simulink model "model_steadystate_pmsm"  (R2022a)
settings: Solver=ode4  StartTime=0.0  StopTime=1  FixedStep=1e-4  RelTol=1e-3
PreLoadFcn:
  | P = 2; %number of poles
settings Model: Creator=samee  LastModifiedBy=samee

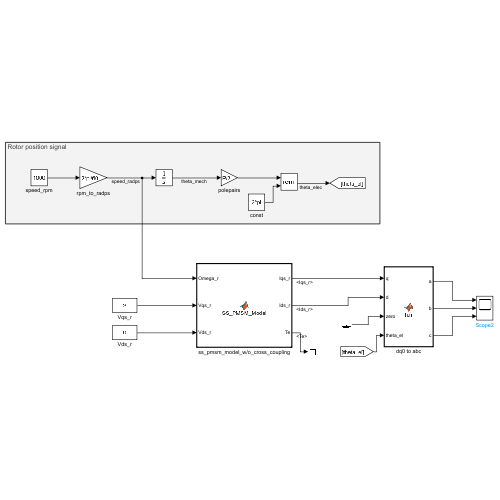
[thumbnail: Simulink's stored preview of the top-level diagram]
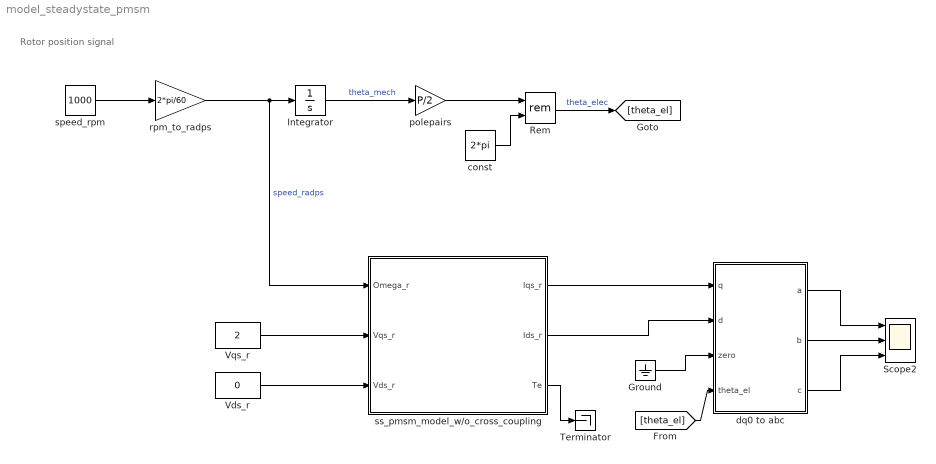
== system model_steadystate_pmsm ==
  note: Rotor position signal
  Ground : Ground
  Integrator : Integrator
  Rem : Math  Operator=rem
  Scope2 : Scope  NumInputPorts=3
  Terminator : Terminator
  Vds_r : Constant  Value=0
  Vqs_r : Constant  Value=2
  const : Constant  Value=2*pi
  dq0 to abc : MATLAB Function  TreatAsAtomicUnit=on
  polepairs : Gain  Gain=P/2
  rpm_to_radps : Gain  Gain=2*pi/60
  speed_rpm : Constant  Value=1000
  ss_pmsm_model_w/o_cross_coupling : MATLAB Function  TreatAsAtomicUnit=on
  wires:
  Integrator/1 -> polepairs/1  "theta_mech"
  const/1 -> Rem/2
  polepairs/1 -> Rem/1
  speed_rpm/1 -> rpm_to_radps/1
  rpm_to_radps/1 -> Integrator/1, ss_pmsm_model_w/o_cross_coupling/1(Omega_r)  "speed_radps"
  Rem/1 -> [theta_el]  "theta_elec"
  Vqs_r/1 -> ss_pmsm_model_w/o_cross_coupling/2(Vqs_r)
  Vds_r/1 -> ss_pmsm_model_w/o_cross_coupling/3(Vds_r)
  ss_pmsm_model_w/o_cross_coupling/1(Iqs_r) -> dq0 to abc/1(q)
  ss_pmsm_model_w/o_cross_coupling/2(Ids_r) -> dq0 to abc/2(d)
  ss_pmsm_model_w/o_cross_coupling/3(Te) -> Terminator/1
  Ground/1 -> dq0 to abc/3(zero)
  dq0 to abc/1(a) -> Scope2/1
  dq0 to abc/2(b) -> Scope2/2
  dq0 to abc/3(c) -> Scope2/3
  [theta_el] -> dq0 to abc/4(theta_el)

== matlab function model_steadystate_pmsm/dq0 to abc ==
  data: q input; d input; a output; zero input; theta_el input; b output; c output
function [a, b, c] = fcn(q, d, zero, theta_el)

a = cos(theta_el)*q + sin(theta_el)*d + zero*1;
b = cos(theta_el-(2*pi/3))*q + sin(theta_el-(2*pi/3))*d + zero*1;
c = cos(theta_el+(2*pi/3))*q + sin(theta_el+(2*pi/3))*d + zero*1;

== matlab function model_steadystate_pmsm/ss_pmsm_model_w//o_cross_coupling ==
  data: Omega_r input; Vqs_r input; Iqs_r output; Vds_r input; Ids_r output; Te output
function [Iqs_r, Ids_r, Te] = SS_PMSM_Model(Omega_r, Vqs_r, Vds_r)
%#codegen

rs = 0.2;               %Stator resistance
Lq = 300e-6;            %d and q axis inductances
Ld = 300e-6;
Lambda_m_r = 0.01;      %rotor flux linkages (back-emf constant)
P=2;                    % numer of poles               


K1 = ((rs^2) + (Omega_r^2)*Ld*Lq);

% Motor currents in rotor reference frame
Iqs_r = (rs/K1) * (Vqs_r - Omega_r*Lambda_m_r - (Omega_r*Ld/rs)*Vds_r);
Ids_r = (1/K1) * (rs*Vds_r + Omega_r*Lq*Vqs_r - (Omega_r^2)*Lq*Lambda_m_r);

% Electromagnetic torque generated
Te = (3/2)*(P/2)*((Lambda_m_r*Iqs_r) + ((Ld - Lq)*Iqs_r*Ids_r));
